simulink model "guidance"  (R2021a)
settings: Solver=VariableStepAuto  StartTime=0.0  StopTime=inf  RelTol=1e-3
undefined symbols (not defined in the file or in its folder): A_mpc, B_mpc, C_mpc, D_mpc, Discrete, dt, Time, wait
libraries: ctrlSharedLib x1, mpclib x1, drivingscenarioandsensors x1
settings Model: Creator=Adam  LastModifiedBy=Adam

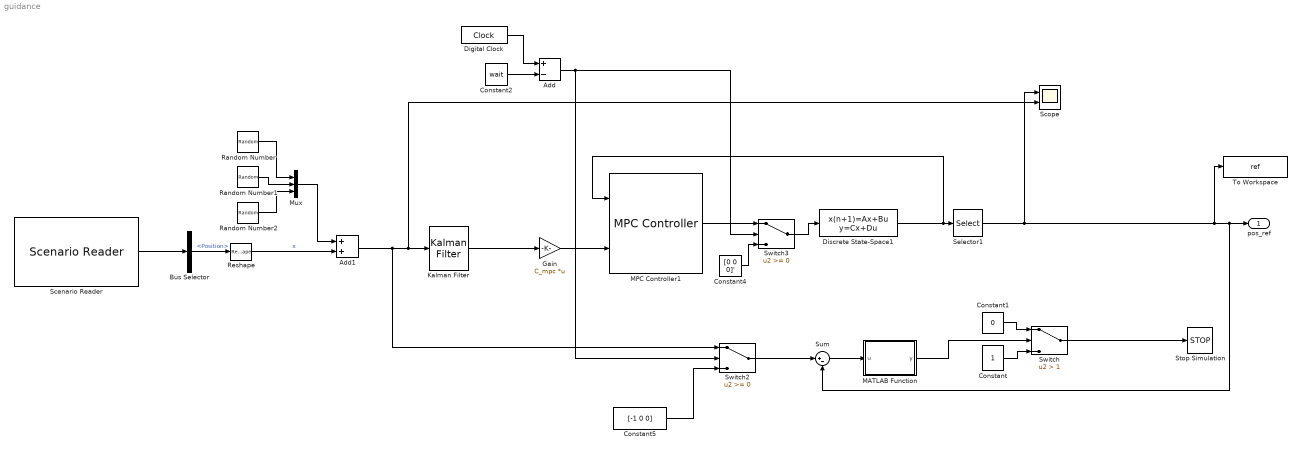
== system guidance ==
  Add : Sum  Inputs=+-
  Add1 : Sum
  Bus Selector : BusSelector  OutputSignals=Actors.Position
  Constant : Constant
  Constant1 : Constant  Value=0
  Constant2 : Constant  Value=wait
  Constant4 : Constant  Value=[0 0 0]'
  Constant5 : Constant  Value=[-1 0 0]
  Digital Clock : DigitalClock  SampleTime=0.01
  Discrete State-Space1 : DiscreteStateSpace  A=A_mpc  B=B_mpc  C=C_mpc  D=D_mpc  InitialCondition="[0;0;0; 0;0;0  ; 5 ;0;0]"  SampleTime=0.01
  Gain : Gain  Gain=C_mpc  Multiplication=Matrix(K*u)
  Kalman Filter : ctrlSharedLib/Kalman Filter  TimeDomain=Discrete-Time  UseCurrentEstimator=on  ModelSource=Individual A, B, C, D matrices  ModelSourceVariable=ss(0.95,1,1,0,1)  A=blkdiag([1 dt 0.5*dt^2;0 1 dt;0 0 1],[1 dt 0.5*dt^2;0 1 dt;0 0 1],[1 dt 0.5*dt^2;0 1 dt;0 0 1])  B=zeros(  C=[1 zeros(1,8); 0 0 0 1 zeros(1,5); zeros(1,6) 1 0 0]  D=0  NumberOfStates=1  NumberOfInputs=1  NumberOfOutputs=1  InitialEstimateSource=Dialog  X0=zeros(9,1)  P0=10  UseK=off  UseGH=on  NumberOfProcessNoiseInputs=1  G=eye(9)  TimeInvariantG=on  H=0  TimeInvariantH=on  Q=eye(9)*0.01  TimeInvariantQ=on  R=eye(3)*0.01  TimeInvariantR=on  N=0  TimeInvariantN=on  AddInputPort=off  AddEnablePort=off  OutputEstimatedY=off  OutputP=off  Ts=0.01
  MATLAB Function : MATLAB Function  TreatAsAtomicUnit=on
  MPC Controller1 : mpclib/MPC Controller  SCDEnableBlockLinearizationSpecification=on  mpcobj=mpc1  is_multiple=0  enable_value=0  return_u0=off  updateMPCinCallerWorkspace=on  md_inport=off  mv_inport=off  uref_inport=off  return_cost=off  return_mvseq=off  return_qpstatus=off  return_xseq=off  return_state=off  return_ovseq=off  state_inport=off  umin_inport=off  umax_inport=off  ymin_inport=off  ymax_inport=off  cc_inport=off  ywt_inport=off  uwt_inport=off  duwt_inport=off  rhoeps_inport=off  pm_inport=off  MaximumP=10  HorizonChoice=FixedHorizon  n_ts=0.01  n_p=10  n_mv=3  n_md=0  n_ud=0  n_mo=9  n_uo=0  BlockDataType=double  SampleTimeInherited=off  switch_inport=off
  Mux : Mux  Inputs=3
  Random Number : RandomNumber  Variance=0.01  SampleTime=0.01  VectorParams1D=off
  Random Number1 : RandomNumber  Variance=0.01  SampleTime=0.01  VectorParams1D=off
  Random Number2 : RandomNumber  Variance=0.01  SampleTime=0.01  VectorParams1D=off
  Reshape : Reshape
  Scenario Reader : drivingscenarioandsensors/Scenario Reader  ScenarioSource=From file  ScenarioFileName=C:\Users\Adam\OneDrive\Desktop\M.Sc_LRT\4.sem\session2\Stage\sim\Scenarios\scenario3.mat  ScenarioVariableName=scenario  OutputCoordinateSystem=World coordinates  EgoVehicleSource=Scenario  EgoVehicleActorID=1  OrientVehiclesOnRoad=off  OutputEgoVehiclePose=off  SampleTime=0.01  LaneBoundaryOutput=None  LaneBoundaryDistance=0:0.5:9.5  LaneBoundaryLocation=Center of lane markings  BusNameSource=Auto  BusName=BusActors  BusNumActorsSource=Scenario  BusNumActors=100  BusName2Source=Auto  BusName2=BusLaneBoundaries  BusNumLaneBoundariesSource=Scenario  BusNumLaneBoundaries=10  BusName3Source=Auto  BusName3=BusEgoActor  ShowCoordinateLabels=on  SimulateUsing=Interpreted execution
  Scope : Scope  NumInputPorts=2
  Selector1 : Selector  InputPortWidth=9  IndexOptions=Index vector (dialog)  Indices=[1 2 3]  OutputSizes=1
  Stop Simulation : Stop
  Sum : Sum  Inputs=|+-
  Switch : Switch  Criteria=u2 > Threshold  Threshold=1
  Switch2 : Switch
  Switch3 : Switch
  To Workspace : ToWorkspace  VariableName=ref  SampleTime=-1
  pos_ref : Outport
  wires:
  Selector1/1 -> Scope/1, To Workspace/1, Sum/2, pos_ref/1
  Switch/1 -> Stop Simulation/1
  Sum/1 -> MATLAB Function/1(u)
  Constant1/1 -> Switch/1
  MATLAB Function/1(y) -> Switch/2
  Constant/1 -> Switch/3
  Discrete State-Space1/1 -> MPC Controller1/1, Selector1/1
  Gain/1 -> MPC Controller1/2
  Scenario Reader/1 -> Bus Selector/1
  Bus Selector/1 -> Reshape/1  "<Position>"
  Digital Clock/1 -> Add/1
  Constant2/1 -> Add/2
  Add/1 -> Switch2/2, Switch3/2
  Constant4/1 -> Switch3/3
  MPC Controller1/1 -> Switch3/1
  Switch3/1 -> Discrete State-Space1/1
  Switch2/1 -> Sum/1
  Reshape/1 -> Add1/2  "x"
  Constant5/1 -> Switch2/3
  Kalman Filter/1 -> Gain/1
  Random Number/1 -> Mux/1
  Random Number1/1 -> Mux/2
  Random Number2/1 -> Mux/3
  Mux/1 -> Add1/1
  Add1/1 -> Switch2/1, Scope/2, Kalman Filter/1

== matlab function guidance/MATLAB Function ==
  data: u input; y output
function y = fcn(u)

y = norm(u);
